simulink model "Model_HVAC_old_controller"  (R2019b)
settings: Solver=VariableStepAuto  StartTime=0.0  StopTime=365*24  RelTol=1e-3
undefined symbols (not defined in the file or in its folder): sigbuilder_block, T_s_in
libraries: simulink x1
(part 2 of 2)

== system Model_HVAC_old_controller/Solar thermal storage/Lower part 3/Storage Area ==
  Add1 : Sum
  Area1 : Display
  Constant : Constant  Value=0.5
  Divide1 : Product  Inputs=***
  Divide2 : Product  Inputs=***
  Math Function : Math  Operator=square  SaturateOnIntegerOverflow=on
  pi : Constant  Value=pi
  Area : Outport  VectorParamsAs1DForOutWhenUnconnected=off
  wires:
  Add1/1 -> Area/1, Area1/1
  [H_s] -> Divide1/1
  pi/1 -> Divide1/2, Divide2/2
  [D_s] -> Divide1/3, Math Function/1
  Math Function/1 -> Divide2/1
  Constant/1 -> Divide2/3
  Divide1/1 -> Add1/1
  Divide2/1 -> Add1/2

== system Model_HVAC_old_controller/Back-up/Prova back-up/Controller Qbu/If Action Subsystem ==
  Action Port : ActionPort  ActionPortLabel=if(u1>=u2)
  Constant : Constant  Value=0
  Out1 : Outport  VectorParamsAs1DForOutWhenUnconnected=off
  wires:
  Constant/1 -> Out1/1

== system Model_HVAC_old_controller/Back-up/Prova back-up/Controller Qbu/If Action Subsystem3 ==
  In1 : Inport
  Action Port : ActionPort  ActionPortLabel=else
  Out1 : Outport  VectorParamsAs1DForOutWhenUnconnected=off
  wires:
  In1/1 -> Out1/1

== system Model_HVAC_old_controller/Solar thermal storage/Lower part 3/Heat Exchanger/Controller Tuhe ==
  Tupump : Inport
  T3 : Inport  Port=2
  Add1 : Sum
  Add4 : Sum  Inputs=+-
  Divide1 : Product  Inputs=**
  Fcn : Fcn  Expr=exp((-u[1])/(u[2]*u[3]))
  Mux : Mux  Inputs=3
  Scope1 : Scope
  Scope2 : Scope
  Scope8 : Scope
  Switch1 : Switch  Criteria=u2 > Threshold  ZeroCross=off
  Tuhe : Outport  VectorParamsAs1DForOutWhenUnconnected=off
  wires:
  Tupump/1 -> Add4/1, Scope2/1
  [Total_fluid_mass] -> Mux/3
  Mux/1 -> Fcn/1
  Add4/1 -> Divide1/1
  Fcn/1 -> Divide1/2
  Divide1/1 -> Add1/2, Scope8/1
  T3/1 -> Add4/2, Add1/1
  Add1/1 -> Switch1/1
  Switch1/1 -> Tuhe/1, Scope1/1
  [Pelpump] -> Switch1/2
  [Tucoll] -> Switch1/3
  [UA_s_ex] -> Mux/1
  [Cp_brine] -> Mux/2

== system Model_HVAC_old_controller/Solar thermal storage/Lower part 3/Heat Exchanger/Integral Block ==
  Watt : Inport
  Integrator : Integrator
  J to MJ : Gain  Gain=1/1000000
  MJ to kWh : Gain  Gain=1/3.6
  MJ1 : Display
  Scope1 : Scope
  Scope2 : Scope
  kWh1 : Display
  MJ : Outport  VectorParamsAs1DForOutWhenUnconnected=off
  kWh : Outport  Port=2  VectorParamsAs1DForOutWhenUnconnected=off
  wires:
  Integrator/1 -> J to MJ/1
  Watt/1 -> Integrator/1
  J to MJ/1 -> Scope1/1, MJ1/1, MJ/1, MJ to kWh/1
  MJ to kWh/1 -> Scope2/1, kWh1/1, kWh/1

== system Model_HVAC_old_controller/Solar thermal storage/Lower part 3/Heat Exchanger/Security System1 ==
  Qsol1 : Inport
  Add1 : Sum  Inputs=+-
  Add2 : Sum  Inputs=+-
  Constant : Constant  Value=0
  Switch : Switch  Criteria=u2 > Threshold  ZeroCross=off
  Switch1 : Switch  Criteria=u2 > Threshold  ZeroCross=off
  Qsol : Outport  VectorParamsAs1DForOutWhenUnconnected=off
  wires:
  Add1/1 -> Switch/2
  Constant/1 -> Switch/3, Switch1/3
  [T_s_max] -> Add1/1
  [T3] -> Add1/2
  Qsol1/1 -> Switch/1
  [Tupump] -> Add2/1
  [T3] -> Add2/2
  Add2/1 -> Switch1/2
  Switch/1 -> Switch1/1
  Switch1/1 -> Qsol/1

== system Model_HVAC_old_controller/Solar thermal storage/Lower part 3/Qgain/Controller Qgain ==
  Qwhr : Inport
  Qsol : Inport  Port=2
  If : If  NumInputs=2  IfExpression=u2<0  ElseIfExpressions=u2>=u1,u2<u1  ShowElse=off  ZeroCross=off
  If Action Subsystem : Subsystem  TreatAsAtomicUnit=on
  If Action Subsystem1 : Subsystem  TreatAsAtomicUnit=on
  If Action Subsystem3 : Subsystem  TreatAsAtomicUnit=on
  Merge : Merge  Inputs=3
  Qstored : Subsystem
  Qgain : Outport  VectorParamsAs1DForOutWhenUnconnected=off
  wires:
  Qwhr/1 -> If/1, If Action Subsystem1/1(In1)
  If/1 -> If Action Subsystem/Action
  If Action Subsystem/1(Out1) -> Merge/1
  If Action Subsystem1/1(Out1) -> Merge/2
  If Action Subsystem3/1(Out1) -> Merge/3
  If/2 -> If Action Subsystem1/Action
  If/3 -> If Action Subsystem3/Action
  Qstored/1(Qstored) -> If/2, If Action Subsystem3/1(In1)
  Qsol/1 -> Qgain/1

== system Model_HVAC_old_controller/Solar thermal storage/Lower part 3/Qgain/Integral Block ==
  Watt : Inport
  Integrator : Integrator
  J to MJ : Gain  Gain=1/1000000
  MJ to kWh : Gain  Gain=1/3.6
  MJ1 : Display
  Scope1 : Scope
  Scope2 : Scope
  kWh1 : Display
  MJ : Outport  VectorParamsAs1DForOutWhenUnconnected=off
  kWh : Outport  Port=2  VectorParamsAs1DForOutWhenUnconnected=off
  wires:
  Integrator/1 -> J to MJ/1
  Watt/1 -> Integrator/1
  J to MJ/1 -> Scope1/1, MJ1/1, MJ/1, MJ to kWh/1
  MJ to kWh/1 -> Scope2/1, kWh1/1, kWh/1

== system Model_HVAC_old_controller/Solar thermal storage/Lower part 3/Qgain/Controller Qgain/If Action Subsystem ==
  Action Port : ActionPort  ActionPortLabel=if(u2<0)
  J to MJ : Constant  Value=0
  Out1 : Outport  VectorParamsAs1DForOutWhenUnconnected=off
  wires:
  J to MJ/1 -> Out1/1

== system Model_HVAC_old_controller/Solar thermal storage/Lower part 3/Qgain/Controller Qgain/If Action Subsystem1 ==
  In1 : Inport
  Action Port : ActionPort  ActionPortLabel=elseif(u2>=u1)
  Out1 : Outport  VectorParamsAs1DForOutWhenUnconnected=off
  wires:
  In1/1 -> Out1/1

== system Model_HVAC_old_controller/Solar thermal storage/Lower part 3/Qgain/Controller Qgain/If Action Subsystem3 ==
  In1 : Inport
  Action Port : ActionPort  ActionPortLabel=elseif(u2<u1)
  Out1 : Outport  VectorParamsAs1DForOutWhenUnconnected=off
  wires:
  In1/1 -> Out1/1

== system Model_HVAC_old_controller/Solar thermal storage/Lower part 3/Qgain/Controller Qgain/Qstored ==
  Add2 : Sum  Inputs=-+
  Product3 : Product  Inputs=***  SaturateOnIntegerOverflow=on  OutDataTypeStr=Inherit: Same as first input
  Qstored : Outport  VectorParamsAs1DForOutWhenUnconnected=off
  wires:
  Product3/1 -> Qstored/1
  [T_acq] -> Add2/1
  [T3] -> Add2/2
  Add2/1 -> Product3/1
  [m] -> Product3/2
  [Cp_water] -> Product3/3
